simulink model "toplevel"  (R2018b)
settings: Solver=FixedStepDiscrete  StartTime=0.0  StopTime=1.0  FixedStep=0.01  RelTol=1e-3
libraries: EdgeCounter x1
settings Model: Creator=moritahiromitsu  LastModifiedBy=moritahiromitsu

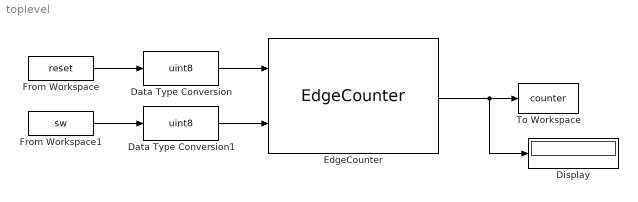
== system toplevel ==
  Data Type Conversion : DataTypeConversion  OutDataTypeStr=uint8  RndMeth=Round  SaturateOnIntegerOverflow=on
  Data Type Conversion1 : DataTypeConversion  OutDataTypeStr=uint8  RndMeth=Nearest  SaturateOnIntegerOverflow=on
  Display : Display
  EdgeCounter : EdgeCounter/EdgeCounter  SystemSampleTime=-1
  From Workspace : FromWorkspace  VariableName=reset  SampleTime=0
  From Workspace1 : FromWorkspace  VariableName=sw  SampleTime=0
  To Workspace : ToWorkspace  VariableName=counter  SaveFormat=Timeseries  SampleTime=-1
  wires:
  From Workspace/1 -> Data Type Conversion/1
  From Workspace1/1 -> Data Type Conversion1/1
  Data Type Conversion/1 -> EdgeCounter/1
  Data Type Conversion1/1 -> EdgeCounter/2
  EdgeCounter/1 -> Display/1, To Workspace/1
